simulink model "TestbedModel_v6"  (R2016a)
settings: Solver=ode23tb  StartTime=0.0  StopTime=20  RelTol=1e-3
undefined symbols (not defined in the file): K, Ki, Kp, magnitude, rev_comms_sink, tau
libraries: DAEMOT_Lib x4
(part 2 of 4)

== system TestbedModel_v6/Air Vehicle ==
  In1 : Inport
  In2 : Inport  Port=2
  Bus Creator2 : BusCreator  Inputs=4
  Bus Selector2 : BusSelector  OutputSignals=aspeed,torque
  Data_Sink : Subsystem  LoadFcn=|  InitFcn=|  mask(Data Sink){}
      LoadFcn=|
      | h      = get_param(gcb,'handle');   % Get block handle                           
      | hblock = get(h);     % Parse out handles structure
      | 
      | str = [hblock.Path(numel(bdroot)+2:end), hblock.Name];
      | str(~ismember(str,['A':'Z' 'a':'z' '0':'9' '_'])) = '';                     
      | set_param([gcb, '/global_data_goto'],'GotoTag',['gdata_',str]);
      |                                
      |                                                                                  
      | clear h hblock str
      InitFcn=|
      | h      = get_param(gcb,'handle');   % Get block handle                           
      | hblock = get(h);     % Parse out handles structure
      | 
      | str = [hblock.Path(numel(bdroot)+2:end), hblock.Name];
      | str(~ismember(str,['A':'Z' 'a':'z' '0':'9' '_'])) = '';                     
      | set_param([gcb, '/global_data_goto'],'GotoTag',['gdata_',str]);
      |                                
      |                                                                                  
      | clear h hblock str
      mask help:
      | Input to this block should be a bus signal with named signals.
      |
      | Bus signals sent to this block will be read by the Data Manager.
      | The Data Manager will handle the global routing of signals.
      |
      | This block should be placed under the mask of components.
      settings: CopyFcn=|
      | h      = get_param(gcb,'handle');   % Get block handle
      | hblock = get(h);     % Parse out handles structure
      | 
      | str = [hblock.Path(numel(bdroot)+2:end), hblock.Name];
      | str(~ismember(str,['A':'Z' 'a':'z' '0':'9' '_'])) = '';
      | set_param([gcb, '/global_data_goto'],'GotoTag',['gdata_',str]);
      | 
      | 
      | clear h hblock str
      settings: NameChangeFcn=|
      | h      = get_param(gcb,'handle');   % Get block handle
      | hblock = get(h);     % Parse out handles structure
      | 
      | str = [hblock.Path(numel(bdroot)+2:end), hblock.Name];
      | str(~ismember(str,['A':'Z' 'a':'z' '0':'9' '_'])) = '';
      | set_param([gcb, '/global_data_goto'],'GotoTag',['gdata_',str]);
      | 
      | 
      | clear h hblock str
      mask Display: text(0.25,0.5,'Data Sink')
  Fcn : Fcn  Expr=u(1)*cos(u(2))
  Fcn1 : Fcn  Expr=u(1)*sin(u(2))
  Integrator : Integrator  InitialCondition=v_initial
  Mux : Mux  Inputs=2
  Property : Subsystem
  Sink1 : Subsystem  LoadFcn=rev_comms_sink();  InitFcn=rev_comms_sink();  mask(Sink){}
      mask help: Used for sending data to the upstream component.
      settings: CopyFcn=rev_comms_sink();  NameChangeFcn=rev_comms_sink();
      mask Display: text(0.25,0.5,'Sink')
  Terminator1 : Terminator
  speed : MATLAB Function  TreatAsAtomicUnit=on
  wires:
  Property/1(Props) -> speed/3(props)
  Integrator/1 -> [v], Property/1(v), speed/1(v)
  [tau] -> Sink1/1(In1)
  Bus Selector2/1 -> [omega]  "<aspeed>"
  In1/1 -> Bus Selector2/1
  Bus Selector2/2 -> Terminator1/1  "<torque>"
  [v] -> Bus Creator2/2  "Vehicle Speed [m_s]"
  Bus Creator2/1 -> Data_Sink/1(" ")
  [tau] -> Bus Creator2/1  "Load Torque [Nm]"
  [omega] -> speed/2(omega), Property/2(w)
  speed/1(v_dot) -> Integrator/1
  speed/2(tau) -> [tau]
  [theta] -> speed/4(theta)
  Fcn/1 -> Bus Creator2/3  "Lateral Speed [m_s]"
  Fcn1/1 -> Bus Creator2/4  "Vertical Speed [m_s]"
  Mux/1 -> Fcn1/1, Fcn/1
  [v] -> Mux/1
  [theta] -> Mux/2
  In2/1 -> [theta]

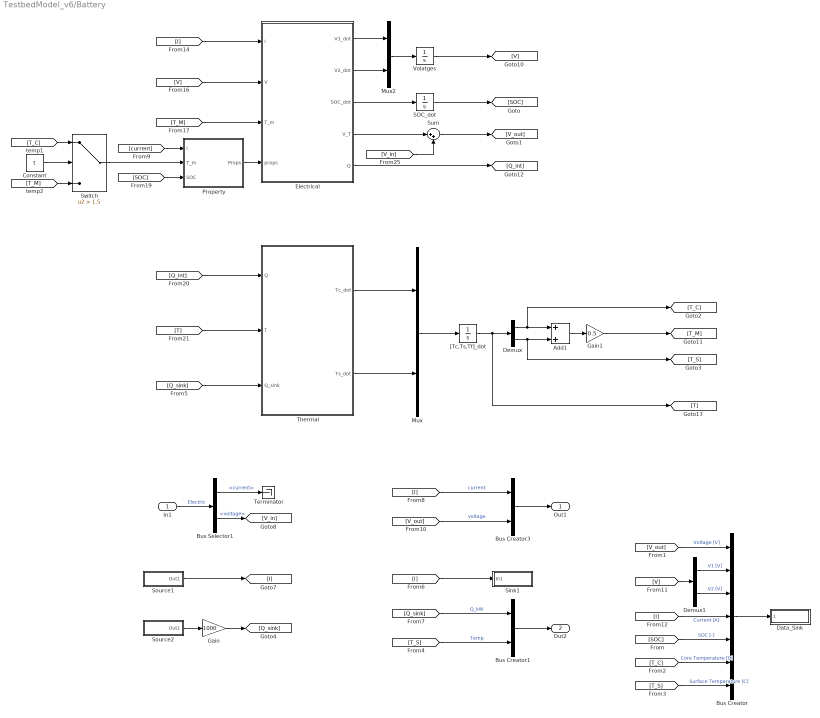
== system TestbedModel_v6/Battery ==
  In1 : Inport
  Add1 : Sum
  Bus Creator : BusCreator  Inputs=7
  Bus Creator1 : BusCreator  Inputs=2
  Bus Creator3 : BusCreator  Inputs=2
  Bus Selector1 : BusSelector  OutputSignals=current,voltage
  Constant : Constant  Value=t
  Data_Sink : Subsystem  LoadFcn=|  InitFcn=|  mask(Data Sink){}
      LoadFcn=|
      | h      = get_param(gcb,'handle');   % Get block handle                           
      | hblock = get(h);     % Parse out handles structure
      | 
      | str = [hblock.Path(numel(bdroot)+2:end), hblock.Name];
      | str(~ismember(str,['A':'Z' 'a':'z' '0':'9' '_'])) = '';                     
      | set_param([gcb, '/global_data_goto'],'GotoTag',['gdata_',str]);
      |                                
      |                                                                                  
      | clear h hblock str
      InitFcn=|
      | h      = get_param(gcb,'handle');   % Get block handle                           
      | hblock = get(h);     % Parse out handles structure
      | 
      | str = [hblock.Path(numel(bdroot)+2:end), hblock.Name];
      | str(~ismember(str,['A':'Z' 'a':'z' '0':'9' '_'])) = '';                     
      | set_param([gcb, '/global_data_goto'],'GotoTag',['gdata_',str]);
      |                                
      |                                                                                  
      | clear h hblock str
      mask help:
      | Input to this block should be a bus signal with named signals.
      |
      | Bus signals sent to this block will be read by the Data Manager.
      | The Data Manager will handle the global routing of signals.
      |
      | This block should be placed under the mask of components.
      settings: CopyFcn=|
      | h      = get_param(gcb,'handle');   % Get block handle
      | hblock = get(h);     % Parse out handles structure
      | 
      | str = [hblock.Path(numel(bdroot)+2:end), hblock.Name];
      | str(~ismember(str,['A':'Z' 'a':'z' '0':'9' '_'])) = '';
      | set_param([gcb, '/global_data_goto'],'GotoTag',['gdata_',str]);
      | 
      | 
      | clear h hblock str
      settings: NameChangeFcn=|
      | h      = get_param(gcb,'handle');   % Get block handle
      | hblock = get(h);     % Parse out handles structure
      | 
      | str = [hblock.Path(numel(bdroot)+2:end), hblock.Name];
      | str(~ismember(str,['A':'Z' 'a':'z' '0':'9' '_'])) = '';
      | set_param([gcb, '/global_data_goto'],'GotoTag',['gdata_',str]);
      | 
      | 
      | clear h hblock str
      mask Display: text(0.25,0.5,'Data Sink')
  Demux : Demux  Outputs=2
  Demux1 : Demux  Outputs=2
  Electrical : MATLAB Function  TreatAsAtomicUnit=on
  Gain : Gain  Gain=1000
  Gain1 : Gain  Gain=0.5
  Mux : Mux  Inputs=2
  Mux2 : Mux  Inputs=2
  Property : Subsystem
  SOC_dot : Integrator  InitialCondition=SOC_initial
  Sink1 : Subsystem  LoadFcn=rev_comms_sink();  InitFcn=rev_comms_sink();  mask(Sink){}
      mask help: Used for sending data to the upstream component.
      settings: CopyFcn=rev_comms_sink();  NameChangeFcn=rev_comms_sink();
      mask Display: text(0.25,0.5,'Sink')
  Source1 : Subsystem  mask(Source){}
      mask help: Used for receiving data from the downstream component.
      mask init:
      | n_src = gcb;
      | n_src = str2num(n_src(end));
      | try
      |     rev_comms_source(n_src);
      | catch
      | 
      | end
      mask Display: text(0.25,0.5,'Source')
  Source2 : Subsystem  mask(Source){}
      mask help: Used for receiving data from the downstream component.
      mask init:
      | n_src = gcb;
      | n_src = str2num(n_src(end));
      | try
      |     rev_comms_source(n_src);
      | catch
      | 
      | end
      mask Display: text(0.25,0.5,'Source')
  Sum : Sum  Inputs=|++
  Switch : Switch  Criteria=u2 > Threshold  Threshold=1.5
  Terminator : Terminator
  Thermal : MATLAB Function  TreatAsAtomicUnit=on
  Volatges : Integrator  InitialCondition=RC_initial
  "[Tc,Ts,Tf]_dot" : Integrator  InitialCondition=[Tc_initial, Ts_initial]
  Out1 : Outport
  Out2 : Outport  Port=2
  wires:
  Gain/1 -> [Q_sink]
  [Q_sink] -> Bus Creator1/1  "Q_kW"
  [T_S] -> Bus Creator1/2  "Temp"
  Bus Creator1/1 -> Out2/1
  Source1/1(Out1) -> [I]
  [I] -> Sink1/1(In1)
  Source2/1(Out1) -> Gain/1
  [Q_sink] -> Thermal/3(Q_sink)
  Thermal/2(Ts_dot) -> Mux/2
  Thermal/1(Tc_dot) -> Mux/1
  [T] -> Thermal/2(T)
  [Q_int] -> Thermal/1(Q)
  [SOC] -> Property/3(SOC)
  Bus Creator/1 -> Data_Sink/1(" ")
  Gain1/1 -> [T_M]
  [current] -> Property/1(I)
  [V_out] -> Bus Creator3/2  "voltage"
  Bus Selector1/2 -> [V_in]  "<voltage>"
  Bus Selector1/1 -> Terminator/1  "<current>"
  [I] -> Bus Creator3/1  "current"
  Bus Creator3/1 -> Out1/1
  In1/1 -> Bus Selector1/1  "Electric"
  [T_S] -> Bus Creator/7  "Surface Temperature [C]"
  [T_C] -> Bus Creator/6  "Core Temperature [C]"
  [V_out] -> Bus Creator/1  "Voltage [V]"
  [SOC] -> Bus Creator/5  "SOC [-]"
  Mux/1 -> "[Tc,Ts,Tf]_dot"/1
  Add1/1 -> Gain1/1
  Volatges/1 -> [V]
  SOC_dot/1 -> [SOC]
  "[Tc,Ts,Tf]_dot"/1 -> Demux/1, [T]
  Demux/1 -> Add1/1, [T_C]
  Demux/2 -> Add1/2, [T_S]
  Mux2/1 -> Volatges/1
  [I] -> Electrical/1(I)
  [T_M] -> Electrical/3(T_m)
  [V] -> Electrical/2(V)
  Property/1(Props) -> Electrical/4(props)
  Electrical/5(Q) -> [Q_int]
  [V_in] -> Sum/2
  Electrical/4(V_T) -> Sum/1
  Sum/1 -> [V_out]
  Electrical/3(SOC_dot) -> SOC_dot/1
  Electrical/1(V1_dot) -> Mux2/1
  Electrical/2(V2_dot) -> Mux2/2
  Constant/1 -> Switch/2
  [T_C] -> Switch/1
  [T_M] -> Switch/3
  Switch/1 -> Property/2(T_m)
  Demux1/2 -> Bus Creator/3  "V2 [V]"
  Demux1/1 -> Bus Creator/2  "V1 [V]"
  [V] -> Demux1/1
  [I] -> Bus Creator/4  "Current [A]"

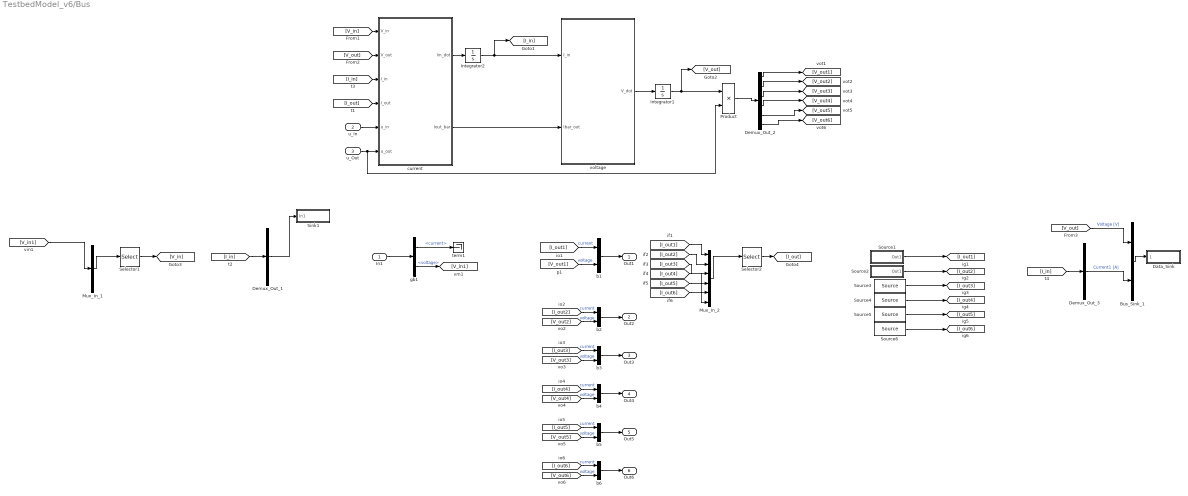
== system TestbedModel_v6/Bus ==
  In1 : Inport
  u_In : Inport  Port=2
  u_Out : Inport  Port=3
  Bus_Sink_1 : BusCreator  Inputs=2
  Data_Sink : Subsystem  LoadFcn=|  InitFcn=|  mask(Data Sink){}
      LoadFcn=|
      | h      = get_param(gcb,'handle');   % Get block handle                           
      | hblock = get(h);     % Parse out handles structure
      | 
      | str = [hblock.Path(numel(bdroot)+2:end), hblock.Name];
      | str(~ismember(str,['A':'Z' 'a':'z' '0':'9' '_'])) = '';                     
      | set_param([gcb, '/global_data_goto'],'GotoTag',['gdata_',str]);
      |                                
      |                                                                                  
      | clear h hblock str
      InitFcn=|
      | h      = get_param(gcb,'handle');   % Get block handle                           
      | hblock = get(h);     % Parse out handles structure
      | 
      | str = [hblock.Path(numel(bdroot)+2:end), hblock.Name];
      | str(~ismember(str,['A':'Z' 'a':'z' '0':'9' '_'])) = '';                     
      | set_param([gcb, '/global_data_goto'],'GotoTag',['gdata_',str]);
      |                                
      |                                                                                  
      | clear h hblock str
      mask help:
      | Input to this block should be a bus signal with named signals.
      |
      | Bus signals sent to this block will be read by the Data Manager.
      | The Data Manager will handle the global routing of signals.
      |
      | This block should be placed under the mask of components.
      settings: CopyFcn=|
      | h      = get_param(gcb,'handle');   % Get block handle
      | hblock = get(h);     % Parse out handles structure
      | 
      | str = [hblock.Path(numel(bdroot)+2:end), hblock.Name];
      | str(~ismember(str,['A':'Z' 'a':'z' '0':'9' '_'])) = '';
      | set_param([gcb, '/global_data_goto'],'GotoTag',['gdata_',str]);
      | 
      | 
      | clear h hblock str
      settings: NameChangeFcn=|
      | h      = get_param(gcb,'handle');   % Get block handle
      | hblock = get(h);     % Parse out handles structure
      | 
      | str = [hblock.Path(numel(bdroot)+2:end), hblock.Name];
      | str(~ismember(str,['A':'Z' 'a':'z' '0':'9' '_'])) = '';
      | set_param([gcb, '/global_data_goto'],'GotoTag',['gdata_',str]);
      | 
      | 
      | clear h hblock str
      mask Display: text(0.25,0.5,'Data Sink')
  Demux_Out_1 : Demux  Outputs=1
  Demux_Out_2 : Demux  Outputs=6
  Demux_Out_3 : Demux  Outputs=1
  Integrator1 : Integrator  InitialCondition=V_initial
  Integrator2 : Integrator  InitialCondition=I_initial*ones(Num_In,1)
  Mux_In_1 : Mux  Inputs=1
  Mux_In_2 : Mux  Inputs=6
  Product : Product
  Selector1 : Selector  InputPortWidth=1  IndexOptions=Index vector (dialog)  Indices=[1 ]  OutputSizes=1
  Selector2 : Selector  InputPortWidth=6  IndexOptions=Index vector (dialog)  Indices=[1 2 3 4 5 6 ]  OutputSizes=1
  Sink1 : Subsystem  LoadFcn=rev_comms_sink();  InitFcn=rev_comms_sink();  mask(Sink){}
      mask help: Used for sending data to the upstream component.
      settings: CopyFcn=rev_comms_sink();  NameChangeFcn=rev_comms_sink();
      mask Display: text(0.25,0.5,'Sink')
  Source1 : Subsystem  mask(Source){}
      mask help: Used for receiving data from the downstream component.
      mask init:
      | n_src = gcb;
      | n_src = str2num(n_src(end));
      | try
      |     rev_comms_source(n_src);
      | catch
      | 
      | end
      mask Display: text(0.25,0.5,'Source')
  Source2 : Subsystem  mask(Source){}
      mask help: Used for receiving data from the downstream component.
      mask init:
      | n_src = gcb;
      | n_src = str2num(n_src(end));
      | try
      |     rev_comms_source(n_src);
      | catch
      | 
      | end
      mask Display: text(0.25,0.5,'Source')
  Source{3..6} (4 alike) : DAEMOT_Lib/Support Functions/Source
  b{1..6} (6 alike) : BusCreator  Inputs=2
  current : MATLAB Function  TreatAsAtomicUnit=on
  gb1 : BusSelector  OutputSignals=current,voltage
  term1 : Terminator
  voltage : MATLAB Function  TreatAsAtomicUnit=on
  Out1 : Outport
  Out2 : Outport  Port=2
  Out3 : Outport  Port=3
  Out4 : Outport  Port=4
  Out5 : Outport  Port=5
  Out6 : Outport  Port=6
  wires:
  Demux_Out_2/2 -> [V_out2]
  [I_out2] -> Mux_In_2/2
  Source2/1(Out1) -> [I_out2]
  b2/1 -> Out2/1
  [V_out2] -> b2/2  "voltage"
  [I_out2] -> b2/1  "current"
  [V_out] -> Bus_Sink_1/1  "Voltage [V]"
  Selector2/1 -> [I_out]
  [I_out] -> current/4(I_out)
  Selector1/1 -> [V_in]
  [V_in] -> current/1(V_in)
  Product/1 -> Demux_Out_2/1
  current/2(Iout_bar) -> voltage/2(Ibar_out)
  u_Out/1 -> current/6(u_out), Product/2
  b1/1 -> Out1/1
  Source1/1(Out1) -> [I_out1]
  [I_out1] -> b1/1  "current"
  [V_out1] -> b1/2  "voltage"
  Mux_In_2/1 -> Selector2/1
  [I_out1] -> Mux_In_2/1
  Bus_Sink_1/1 -> Data_Sink/1(" ")
  Demux_Out_2/1 -> [V_out1]
  u_In/1 -> current/5(u_in)
  [I_in] -> current/3(I_in)
  current/1(Iin_dot) -> Integrator2/1
  Mux_In_1/1 -> Selector1/1
  [V_out] -> current/2(V_out)
  Integrator1/1 -> [V_out], Product/1
  voltage/1(V_dot) -> Integrator1/1
  Integrator2/1 -> [I_in], voltage/1(I_in)
  [I_in] -> Demux_Out_1/1
  In1/1 -> gb1/1
  gb1/1 -> term1/1  "<current>"
  gb1/2 -> [V_in1]  "<voltage>"
  [V_in1] -> Mux_In_1/1
  Demux_Out_1/1 -> Sink1/1(In1)
  [I_in] -> Demux_Out_3/1
  Demux_Out_3/1 -> Bus_Sink_1/2  "Current1 [A]"
  [I_out3] -> b3/1  "current"
  [V_out3] -> b3/2  "voltage"
  b3/1 -> Out3/1
  Source3/1 -> [I_out3]
  [I_out3] -> Mux_In_2/3
  Demux_Out_2/3 -> [V_out3]
  [I_out4] -> b4/1  "current"
  [V_out4] -> b4/2  "voltage"
  b4/1 -> Out4/1
  Source4/1 -> [I_out4]
  [I_out4] -> Mux_In_2/4
  Demux_Out_2/4 -> [V_out4]
  [I_out5] -> b5/1  "current"
  [V_out5] -> b5/2  "voltage"
  b5/1 -> Out5/1
  Source5/1 -> [I_out5]
  [I_out5] -> Mux_In_2/5
  Demux_Out_2/5 -> [V_out5]
  [I_out6] -> b6/1  "current"
  [V_out6] -> b6/2  "voltage"
  b6/1 -> Out6/1
  Source6/1 -> [I_out6]
  [I_out6] -> Mux_In_2/6
  Demux_Out_2/6 -> [V_out6]

== system TestbedModel_v6/Capacitor ==
  In1 : Inport
  Bus Creator1 : BusCreator  Inputs=1
  Bus Creator3 : BusCreator  Inputs=2
  Bus Selector1 : BusSelector  OutputSignals=current,voltage
  Data_Sink : Subsystem  LoadFcn=|  InitFcn=|  mask(Data Sink){}
      LoadFcn=|
      | h      = get_param(gcb,'handle');   % Get block handle                           
      | hblock = get(h);     % Parse out handles structure
      | 
      | str = [hblock.Path(numel(bdroot)+2:end), hblock.Name];
      | str(~ismember(str,['A':'Z' 'a':'z' '0':'9' '_'])) = '';                     
      | set_param([gcb, '/global_data_goto'],'GotoTag',['gdata_',str]);
      |                                
      |                                                                                  
      | clear h hblock str
      InitFcn=|
      | h      = get_param(gcb,'handle');   % Get block handle                           
      | hblock = get(h);     % Parse out handles structure
      | 
      | str = [hblock.Path(numel(bdroot)+2:end), hblock.Name];
      | str(~ismember(str,['A':'Z' 'a':'z' '0':'9' '_'])) = '';                     
      | set_param([gcb, '/global_data_goto'],'GotoTag',['gdata_',str]);
      |                                
      |                                                                                  
      | clear h hblock str
      mask help:
      | Input to this block should be a bus signal with named signals.
      |
      | Bus signals sent to this block will be read by the Data Manager.
      | The Data Manager will handle the global routing of signals.
      |
      | This block should be placed under the mask of components.
      settings: CopyFcn=|
      | h      = get_param(gcb,'handle');   % Get block handle
      | hblock = get(h);     % Parse out handles structure
      | 
      | str = [hblock.Path(numel(bdroot)+2:end), hblock.Name];
      | str(~ismember(str,['A':'Z' 'a':'z' '0':'9' '_'])) = '';
      | set_param([gcb, '/global_data_goto'],'GotoTag',['gdata_',str]);
      | 
      | 
      | clear h hblock str
      settings: NameChangeFcn=|
      | h      = get_param(gcb,'handle');   % Get block handle
      | hblock = get(h);     % Parse out handles structure
      | 
      | str = [hblock.Path(numel(bdroot)+2:end), hblock.Name];
      | str(~ismember(str,['A':'Z' 'a':'z' '0':'9' '_'])) = '';
      | set_param([gcb, '/global_data_goto'],'GotoTag',['gdata_',str]);
      | 
      | 
      | clear h hblock str
      mask Display: text(0.25,0.5,'Data Sink')
  Integrator2 : Integrator  InitialCondition=V_initial
  Sink1 : Subsystem  LoadFcn=rev_comms_sink();  InitFcn=rev_comms_sink();  mask(Sink){}
      mask help: Used for sending data to the upstream component.
      settings: CopyFcn=rev_comms_sink();  NameChangeFcn=rev_comms_sink();
      mask Display: text(0.25,0.5,'Sink')
  Source1 : Subsystem  mask(Source){}
      mask help: Used for receiving data from the downstream component.
      mask init:
      | n_src = gcb;
      | n_src = str2num(n_src(end));
      | try
      |     rev_comms_source(n_src);
      | catch
      | 
      | end
      mask Display: text(0.25,0.5,'Source')
  Terminator : Terminator
  Voltage : MATLAB Function  TreatAsAtomicUnit=on
  Out1 : Outport
  wires:
  Source1/1(Out1) -> [Current_out]
  Bus Creator1/1 -> Data_Sink/1(" ")
  [V] -> Bus Creator1/1  "Voltage [V]"
  [Current_in] -> Voltage/1(I_in)
  Voltage/1(V_dot) -> Integrator2/1
  Bus Creator3/1 -> Out1/1
  [Current_out] -> Voltage/2(I_out)
  In1/1 -> Bus Selector1/1  "electric"
  [V] -> Sink1/1(In1)
  [V] -> Bus Creator3/2  "voltage"
  Bus Selector1/2 -> Terminator/1  "<voltage>"
  Bus Selector1/1 -> [Current_in]  "<current>"
  [Current_out] -> Bus Creator3/1  "current"
  Integrator2/1 -> [V]

== system TestbedModel_v6/Capacitor1 ==
  In1 : Inport
  Bus Creator1 : BusCreator  Inputs=1
  Bus Creator3 : BusCreator  Inputs=2
  Bus Selector1 : BusSelector  OutputSignals=current,voltage
  Data_Sink : Subsystem  LoadFcn=|  InitFcn=|  mask(Data Sink){}
      LoadFcn=|
      | h      = get_param(gcb,'handle');   % Get block handle                           
      | hblock = get(h);     % Parse out handles structure
      | 
      | str = [hblock.Path(numel(bdroot)+2:end), hblock.Name];
      | str(~ismember(str,['A':'Z' 'a':'z' '0':'9' '_'])) = '';                     
      | set_param([gcb, '/global_data_goto'],'GotoTag',['gdata_',str]);
      |                                
      |                                                                                  
      | clear h hblock str
      InitFcn=|
      | h      = get_param(gcb,'handle');   % Get block handle                           
      | hblock = get(h);     % Parse out handles structure
      | 
      | str = [hblock.Path(numel(bdroot)+2:end), hblock.Name];
      | str(~ismember(str,['A':'Z' 'a':'z' '0':'9' '_'])) = '';                     
      | set_param([gcb, '/global_data_goto'],'GotoTag',['gdata_',str]);
      |                                
      |                                                                                  
      | clear h hblock str
      mask help:
      | Input to this block should be a bus signal with named signals.
      |
      | Bus signals sent to this block will be read by the Data Manager.
      | The Data Manager will handle the global routing of signals.
      |
      | This block should be placed under the mask of components.
      settings: CopyFcn=|
      | h      = get_param(gcb,'handle');   % Get block handle
      | hblock = get(h);     % Parse out handles structure
      | 
      | str = [hblock.Path(numel(bdroot)+2:end), hblock.Name];
      | str(~ismember(str,['A':'Z' 'a':'z' '0':'9' '_'])) = '';
      | set_param([gcb, '/global_data_goto'],'GotoTag',['gdata_',str]);
      | 
      | 
      | clear h hblock str
      settings: NameChangeFcn=|
      | h      = get_param(gcb,'handle');   % Get block handle
      | hblock = get(h);     % Parse out handles structure
      | 
      | str = [hblock.Path(numel(bdroot)+2:end), hblock.Name];
      | str(~ismember(str,['A':'Z' 'a':'z' '0':'9' '_'])) = '';
      | set_param([gcb, '/global_data_goto'],'GotoTag',['gdata_',str]);
      | 
      | 
      | clear h hblock str
      mask Display: text(0.25,0.5,'Data Sink')
  Integrator2 : Integrator  InitialCondition=V_initial
  Sink1 : Subsystem  LoadFcn=rev_comms_sink();  InitFcn=rev_comms_sink();  mask(Sink){}
      mask help: Used for sending data to the upstream component.
      settings: CopyFcn=rev_comms_sink();  NameChangeFcn=rev_comms_sink();
      mask Display: text(0.25,0.5,'Sink')
  Source1 : Subsystem  mask(Source){}
      mask help: Used for receiving data from the downstream component.
      mask init:
      | n_src = gcb;
      | n_src = str2num(n_src(end));
      | try
      |     rev_comms_source(n_src);
      | catch
      | 
      | end
      mask Display: text(0.25,0.5,'Source')
  Terminator : Terminator
  Voltage : MATLAB Function  TreatAsAtomicUnit=on
  Out1 : Outport
  wires:
  Integrator2/1 -> [V]
  [Current_out] -> Bus Creator3/1  "current"
  Bus Selector1/1 -> [Current_in]  "<current>"
  Bus Selector1/2 -> Terminator/1  "<voltage>"
  [V] -> Bus Creator3/2  "voltage"
  [V] -> Sink1/1(In1)
  In1/1 -> Bus Selector1/1  "electric"
  [Current_out] -> Voltage/2(I_out)
  Bus Creator3/1 -> Out1/1
  Voltage/1(V_dot) -> Integrator2/1
  [Current_in] -> Voltage/1(I_in)
  [V] -> Bus Creator1/1  "Voltage [V]"
  Bus Creator1/1 -> Data_Sink/1(" ")
  Source1/1(Out1) -> [Current_out]

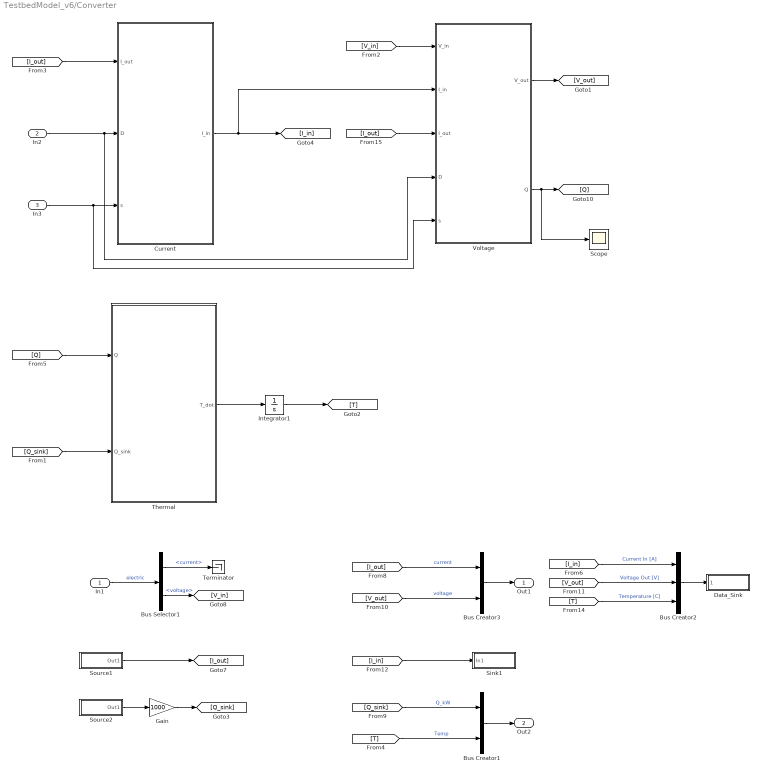
== system TestbedModel_v6/Converter ==
  In1 : Inport
  In2 : Inport  Port=2
  In3 : Inport  Port=3
  Bus Creator1 : BusCreator  Inputs=2
  Bus Creator2 : BusCreator  Inputs=3
  Bus Creator3 : BusCreator  Inputs=2
  Bus Selector1 : BusSelector  OutputSignals=current,voltage
  Current : MATLAB Function  TreatAsAtomicUnit=on
  Data_Sink : Subsystem  LoadFcn=|  InitFcn=|  mask(Data Sink){}
      LoadFcn=|
      | h      = get_param(gcb,'handle');   % Get block handle                           
      | hblock = get(h);     % Parse out handles structure
      | 
      | str = [hblock.Path(numel(bdroot)+2:end), hblock.Name];
      | str(~ismember(str,['A':'Z' 'a':'z' '0':'9' '_'])) = '';                     
      | set_param([gcb, '/global_data_goto'],'GotoTag',['gdata_',str]);
      |                                
      |                                                                                  
      | clear h hblock str
      InitFcn=|
      | h      = get_param(gcb,'handle');   % Get block handle                           
      | hblock = get(h);     % Parse out handles structure
      | 
      | str = [hblock.Path(numel(bdroot)+2:end), hblock.Name];
      | str(~ismember(str,['A':'Z' 'a':'z' '0':'9' '_'])) = '';                     
      | set_param([gcb, '/global_data_goto'],'GotoTag',['gdata_',str]);
      |                                
      |                                                                                  
      | clear h hblock str
      mask help:
      | Input to this block should be a bus signal with named signals.
      |
      | Bus signals sent to this block will be read by the Data Manager.
      | The Data Manager will handle the global routing of signals.
      |
      | This block should be placed under the mask of components.
      settings: CopyFcn=|
      | h      = get_param(gcb,'handle');   % Get block handle
      | hblock = get(h);     % Parse out handles structure
      | 
      | str = [hblock.Path(numel(bdroot)+2:end), hblock.Name];
      | str(~ismember(str,['A':'Z' 'a':'z' '0':'9' '_'])) = '';
      | set_param([gcb, '/global_data_goto'],'GotoTag',['gdata_',str]);
      | 
      | 
      | clear h hblock str
      settings: NameChangeFcn=|
      | h      = get_param(gcb,'handle');   % Get block handle
      | hblock = get(h);     % Parse out handles structure
      | 
      | str = [hblock.Path(numel(bdroot)+2:end), hblock.Name];
      | str(~ismember(str,['A':'Z' 'a':'z' '0':'9' '_'])) = '';
      | set_param([gcb, '/global_data_goto'],'GotoTag',['gdata_',str]);
      | 
      | 
      | clear h hblock str
      mask Display: text(0.25,0.5,'Data Sink')
  Gain : Gain  Gain=1000
  Integrator1 : Integrator  InitialCondition=T_initial
  Scope : Scope
  Sink1 : Subsystem  LoadFcn=rev_comms_sink();  InitFcn=rev_comms_sink();  mask(Sink){}
      mask help: Used for sending data to the upstream component.
      settings: CopyFcn=rev_comms_sink();  NameChangeFcn=rev_comms_sink();
      mask Display: text(0.25,0.5,'Sink')
  Source1 : Subsystem  mask(Source){}
      mask help: Used for receiving data from the downstream component.
      mask init:
      | n_src = gcb;
      | n_src = str2num(n_src(end));
      | try
      |     rev_comms_source(n_src);
      | catch
      | 
      | end
      mask Display: text(0.25,0.5,'Source')
  Source2 : Subsystem  mask(Source){}
      mask help: Used for receiving data from the downstream component.
      mask init:
      | n_src = gcb;
      | n_src = str2num(n_src(end));
      | try
      |     rev_comms_source(n_src);
      | catch
      | 
      | end
      mask Display: text(0.25,0.5,'Source')
  Terminator : Terminator
  Thermal : MATLAB Function  TreatAsAtomicUnit=on
  Voltage : MATLAB Function  TreatAsAtomicUnit=on
  Out1 : Outport
  Out2 : Outport  Port=2
  wires:
  Source2/1(Out1) -> Gain/1
  Voltage/2(Q) -> Scope/1, [Q]
  [I_out] -> Voltage/3(I_out)
  [T] -> Bus Creator2/3  "Temperature [C]"
  [I_in] -> Bus Creator2/1  "Current In [A]"
  [V_out] -> Bus Creator2/2  "Voltage Out [V]"
  Bus Creator2/1 -> Data_Sink/1(" ")
  Thermal/1(T_dot) -> Integrator1/1
  Integrator1/1 -> [T]
  [Q] -> Thermal/1(Q)
  [Q_sink] -> Thermal/2(Q_sink)
  In3/1 -> Current/3(s), Voltage/5(s)
  In2/1 -> Current/2(D), Voltage/4(D)
  Current/1(I_in) -> [I_in], Voltage/2(I_in)
  [I_out] -> Current/1(I_out)
  Voltage/1(V_out) -> [V_out]
  [V_in] -> Voltage/1(V_in)
  [I_out] -> Bus Creator3/1  "current"
  Source1/1(Out1) -> [I_out]
  Bus Selector1/1 -> Terminator/1  "<current>"
  Bus Selector1/2 -> [V_in]  "<voltage>"
  [V_out] -> Bus Creator3/2  "voltage"
  In1/1 -> Bus Selector1/1  "electric"
  Bus Creator3/1 -> Out1/1
  [I_in] -> Sink1/1(In1)
  Bus Creator1/1 -> Out2/1
  [T] -> Bus Creator1/2  "Temp"
  [Q_sink] -> Bus Creator1/1  "Q_kW"
  Gain/1 -> [Q_sink]

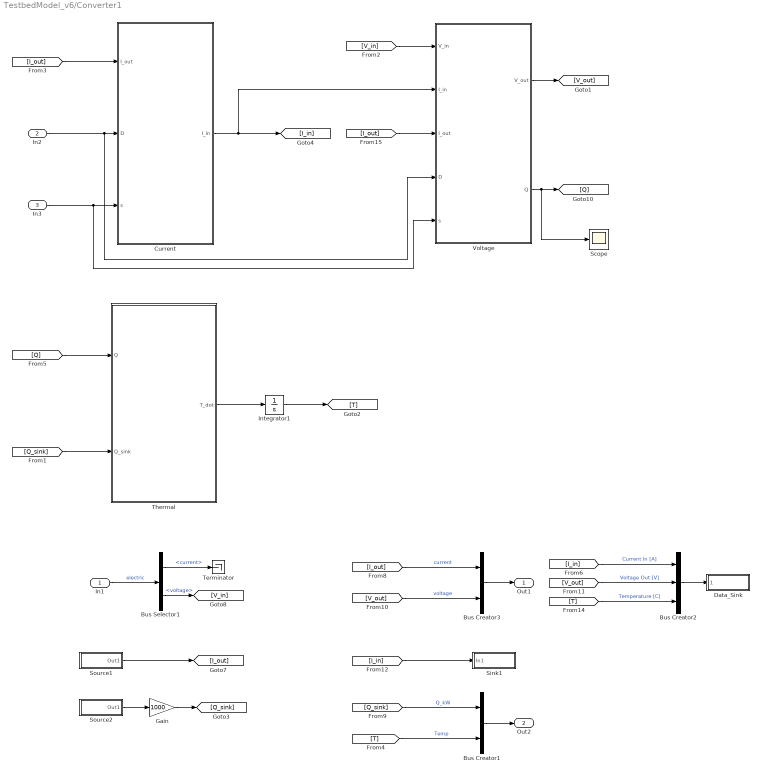
== system TestbedModel_v6/Converter1 ==
  In1 : Inport
  In2 : Inport  Port=2
  In3 : Inport  Port=3
  Bus Creator1 : BusCreator  Inputs=2
  Bus Creator2 : BusCreator  Inputs=3
  Bus Creator3 : BusCreator  Inputs=2
  Bus Selector1 : BusSelector  OutputSignals=current,voltage
  Current : MATLAB Function  TreatAsAtomicUnit=on
  Data_Sink : Subsystem  LoadFcn=|  InitFcn=|  mask(Data Sink){}
      LoadFcn=|
      | h      = get_param(gcb,'handle');   % Get block handle                           
      | hblock = get(h);     % Parse out handles structure
      | 
      | str = [hblock.Path(numel(bdroot)+2:end), hblock.Name];
      | str(~ismember(str,['A':'Z' 'a':'z' '0':'9' '_'])) = '';                     
      | set_param([gcb, '/global_data_goto'],'GotoTag',['gdata_',str]);
      |                                
      |                                                                                  
      | clear h hblock str
      InitFcn=|
      | h      = get_param(gcb,'handle');   % Get block handle                           
      | hblock = get(h);     % Parse out handles structure
      | 
      | str = [hblock.Path(numel(bdroot)+2:end), hblock.Name];
      | str(~ismember(str,['A':'Z' 'a':'z' '0':'9' '_'])) = '';                     
      | set_param([gcb, '/global_data_goto'],'GotoTag',['gdata_',str]);
      |                                
      |                                                                                  
      | clear h hblock str
      mask help:
      | Input to this block should be a bus signal with named signals.
      |
      | Bus signals sent to this block will be read by the Data Manager.
      | The Data Manager will handle the global routing of signals.
      |
      | This block should be placed under the mask of components.
      settings: CopyFcn=|
      | h      = get_param(gcb,'handle');   % Get block handle
      | hblock = get(h);     % Parse out handles structure
      | 
      | str = [hblock.Path(numel(bdroot)+2:end), hblock.Name];
      | str(~ismember(str,['A':'Z' 'a':'z' '0':'9' '_'])) = '';
      | set_param([gcb, '/global_data_goto'],'GotoTag',['gdata_',str]);
      | 
      | 
      | clear h hblock str
      settings: NameChangeFcn=|
      | h      = get_param(gcb,'handle');   % Get block handle
      | hblock = get(h);     % Parse out handles structure
      | 
      | str = [hblock.Path(numel(bdroot)+2:end), hblock.Name];
      | str(~ismember(str,['A':'Z' 'a':'z' '0':'9' '_'])) = '';
      | set_param([gcb, '/global_data_goto'],'GotoTag',['gdata_',str]);
      | 
      | 
      | clear h hblock str
      mask Display: text(0.25,0.5,'Data Sink')
  Gain : Gain  Gain=1000
  Integrator1 : Integrator  InitialCondition=T_initial
  Scope : Scope
  Sink1 : Subsystem  LoadFcn=rev_comms_sink();  InitFcn=rev_comms_sink();  mask(Sink){}
      mask help: Used for sending data to the upstream component.
      settings: CopyFcn=rev_comms_sink();  NameChangeFcn=rev_comms_sink();
      mask Display: text(0.25,0.5,'Sink')
  Source1 : Subsystem  mask(Source){}
      mask help: Used for receiving data from the downstream component.
      mask init:
      | n_src = gcb;
      | n_src = str2num(n_src(end));
      | try
      |     rev_comms_source(n_src);
      | catch
      | 
      | end
      mask Display: text(0.25,0.5,'Source')
  Source2 : Subsystem  mask(Source){}
      mask help: Used for receiving data from the downstream component.
      mask init:
      | n_src = gcb;
      | n_src = str2num(n_src(end));
      | try
      |     rev_comms_source(n_src);
      | catch
      | 
      | end
      mask Display: text(0.25,0.5,'Source')
  Terminator : Terminator
  Thermal : MATLAB Function  TreatAsAtomicUnit=on
  Voltage : MATLAB Function  TreatAsAtomicUnit=on
  Out1 : Outport
  Out2 : Outport  Port=2
  wires:
  Gain/1 -> [Q_sink]
  [Q_sink] -> Bus Creator1/1  "Q_kW"
  [T] -> Bus Creator1/2  "Temp"
  Bus Creator1/1 -> Out2/1
  [I_in] -> Sink1/1(In1)
  Bus Creator3/1 -> Out1/1
  In1/1 -> Bus Selector1/1  "electric"
  [V_out] -> Bus Creator3/2  "voltage"
  Bus Selector1/2 -> [V_in]  "<voltage>"
  Bus Selector1/1 -> Terminator/1  "<current>"
  Source1/1(Out1) -> [I_out]
  [I_out] -> Bus Creator3/1  "current"
  [V_in] -> Voltage/1(V_in)
  Voltage/1(V_out) -> [V_out]
  [I_out] -> Current/1(I_out)
  Current/1(I_in) -> Voltage/2(I_in), [I_in]
  In2/1 -> Voltage/4(D), Current/2(D)
  In3/1 -> Voltage/5(s), Current/3(s)
  [Q_sink] -> Thermal/2(Q_sink)
  [Q] -> Thermal/1(Q)
  Integrator1/1 -> [T]
  Thermal/1(T_dot) -> Integrator1/1
  Bus Creator2/1 -> Data_Sink/1(" ")
  [V_out] -> Bus Creator2/2  "Voltage Out [V]"
  [I_in] -> Bus Creator2/1  "Current In [A]"
  [T] -> Bus Creator2/3  "Temperature [C]"
  [I_out] -> Voltage/3(I_out)
  Voltage/2(Q) -> [Q], Scope/1
  Source2/1(Out1) -> Gain/1

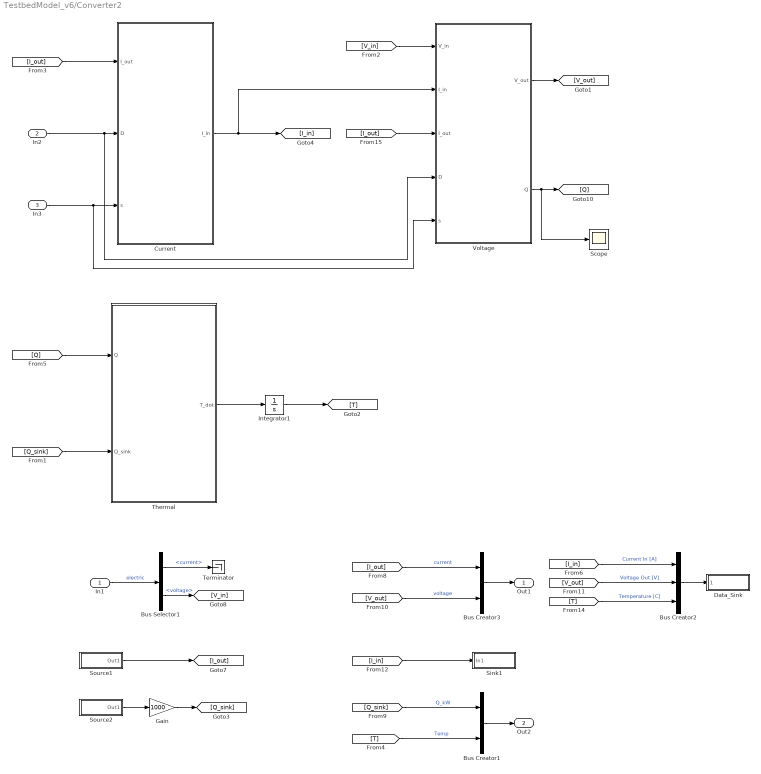
== system TestbedModel_v6/Converter2 ==
  In1 : Inport
  In2 : Inport  Port=2
  In3 : Inport  Port=3
  Bus Creator1 : BusCreator  Inputs=2
  Bus Creator2 : BusCreator  Inputs=3
  Bus Creator3 : BusCreator  Inputs=2
  Bus Selector1 : BusSelector  OutputSignals=current,voltage
  Current : MATLAB Function  TreatAsAtomicUnit=on
  Data_Sink : Subsystem  LoadFcn=|  InitFcn=|  mask(Data Sink){}
      LoadFcn=|
      | h      = get_param(gcb,'handle');   % Get block handle                           
      | hblock = get(h);     % Parse out handles structure
      | 
      | str = [hblock.Path(numel(bdroot)+2:end), hblock.Name];
      | str(~ismember(str,['A':'Z' 'a':'z' '0':'9' '_'])) = '';                     
      | set_param([gcb, '/global_data_goto'],'GotoTag',['gdata_',str]);
      |                                
      |                                                                                  
      | clear h hblock str
      InitFcn=|
      | h      = get_param(gcb,'handle');   % Get block handle                           
      | hblock = get(h);     % Parse out handles structure
      | 
      | str = [hblock.Path(numel(bdroot)+2:end), hblock.Name];
      | str(~ismember(str,['A':'Z' 'a':'z' '0':'9' '_'])) = '';                     
      | set_param([gcb, '/global_data_goto'],'GotoTag',['gdata_',str]);
      |                                
      |                                                                                  
      | clear h hblock str
      mask help:
      | Input to this block should be a bus signal with named signals.
      |
      | Bus signals sent to this block will be read by the Data Manager.
      | The Data Manager will handle the global routing of signals.
      |
      | This block should be placed under the mask of components.
      settings: CopyFcn=|
      | h      = get_param(gcb,'handle');   % Get block handle
      | hblock = get(h);     % Parse out handles structure
      | 
      | str = [hblock.Path(numel(bdroot)+2:end), hblock.Name];
      | str(~ismember(str,['A':'Z' 'a':'z' '0':'9' '_'])) = '';
      | set_param([gcb, '/global_data_goto'],'GotoTag',['gdata_',str]);
      | 
      | 
      | clear h hblock str
      settings: NameChangeFcn=|
      | h      = get_param(gcb,'handle');   % Get block handle
      | hblock = get(h);     % Parse out handles structure
      | 
      | str = [hblock.Path(numel(bdroot)+2:end), hblock.Name];
      | str(~ismember(str,['A':'Z' 'a':'z' '0':'9' '_'])) = '';
      | set_param([gcb, '/global_data_goto'],'GotoTag',['gdata_',str]);
      | 
      | 
      | clear h hblock str
      mask Display: text(0.25,0.5,'Data Sink')
  Gain : Gain  Gain=1000
  Integrator1 : Integrator  InitialCondition=T_initial
  Scope : Scope
  Sink1 : Subsystem  LoadFcn=rev_comms_sink();  InitFcn=rev_comms_sink();  mask(Sink){}
      mask help: Used for sending data to the upstream component.
      settings: CopyFcn=rev_comms_sink();  NameChangeFcn=rev_comms_sink();
      mask Display: text(0.25,0.5,'Sink')
  Source1 : Subsystem  mask(Source){}
      mask help: Used for receiving data from the downstream component.
      mask init:
      | n_src = gcb;
      | n_src = str2num(n_src(end));
      | try
      |     rev_comms_source(n_src);
      | catch
      | 
      | end
      mask Display: text(0.25,0.5,'Source')
  Source2 : Subsystem  mask(Source){}
      mask help: Used for receiving data from the downstream component.
      mask init:
      | n_src = gcb;
      | n_src = str2num(n_src(end));
      | try
      |     rev_comms_source(n_src);
      | catch
      | 
      | end
      mask Display: text(0.25,0.5,'Source')
  Terminator : Terminator
  Thermal : MATLAB Function  TreatAsAtomicUnit=on
  Voltage : MATLAB Function  TreatAsAtomicUnit=on
  Out1 : Outport
  Out2 : Outport  Port=2
  wires:
  Source2/1(Out1) -> Gain/1
  Voltage/2(Q) -> Scope/1, [Q]
  [I_out] -> Voltage/3(I_out)
  [T] -> Bus Creator2/3  "Temperature [C]"
  [I_in] -> Bus Creator2/1  "Current In [A]"
  [V_out] -> Bus Creator2/2  "Voltage Out [V]"
  Bus Creator2/1 -> Data_Sink/1(" ")
  Thermal/1(T_dot) -> Integrator1/1
  Integrator1/1 -> [T]
  [Q] -> Thermal/1(Q)
  [Q_sink] -> Thermal/2(Q_sink)
  In3/1 -> Current/3(s), Voltage/5(s)
  In2/1 -> Current/2(D), Voltage/4(D)
  Current/1(I_in) -> [I_in], Voltage/2(I_in)
  [I_out] -> Current/1(I_out)
  Voltage/1(V_out) -> [V_out]
  [V_in] -> Voltage/1(V_in)
  [I_out] -> Bus Creator3/1  "current"
  Source1/1(Out1) -> [I_out]
  Bus Selector1/1 -> Terminator/1  "<current>"
  Bus Selector1/2 -> [V_in]  "<voltage>"
  [V_out] -> Bus Creator3/2  "voltage"
  In1/1 -> Bus Selector1/1  "electric"
  Bus Creator3/1 -> Out1/1
  [I_in] -> Sink1/1(In1)
  Bus Creator1/1 -> Out2/1
  [T] -> Bus Creator1/2  "Temp"
  [Q_sink] -> Bus Creator1/1  "Q_kW"
  Gain/1 -> [Q_sink]

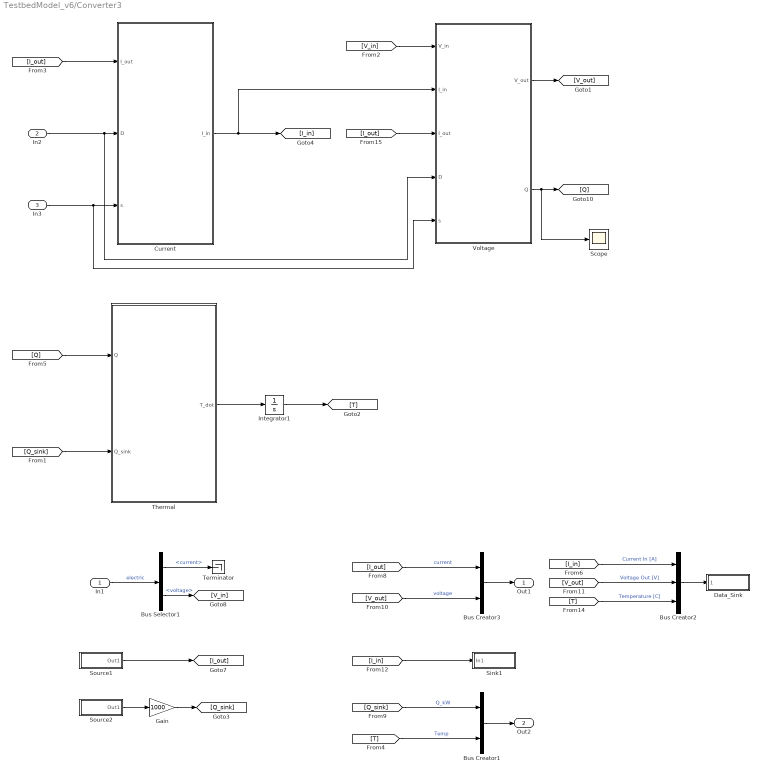
== system TestbedModel_v6/Converter3 ==
  In1 : Inport
  In2 : Inport  Port=2
  In3 : Inport  Port=3
  Bus Creator1 : BusCreator  Inputs=2
  Bus Creator2 : BusCreator  Inputs=3
  Bus Creator3 : BusCreator  Inputs=2
  Bus Selector1 : BusSelector  OutputSignals=current,voltage
  Current : MATLAB Function  TreatAsAtomicUnit=on
  Data_Sink : Subsystem  LoadFcn=|  InitFcn=|  mask(Data Sink){}
      LoadFcn=|
      | h      = get_param(gcb,'handle');   % Get block handle                           
      | hblock = get(h);     % Parse out handles structure
      | 
      | str = [hblock.Path(numel(bdroot)+2:end), hblock.Name];
      | str(~ismember(str,['A':'Z' 'a':'z' '0':'9' '_'])) = '';                     
      | set_param([gcb, '/global_data_goto'],'GotoTag',['gdata_',str]);
      |                                
      |                                                                                  
      | clear h hblock str
      InitFcn=|
      | h      = get_param(gcb,'handle');   % Get block handle                           
      | hblock = get(h);     % Parse out handles structure
      | 
      | str = [hblock.Path(numel(bdroot)+2:end), hblock.Name];
      | str(~ismember(str,['A':'Z' 'a':'z' '0':'9' '_'])) = '';                     
      | set_param([gcb, '/global_data_goto'],'GotoTag',['gdata_',str]);
      |                                
      |                                                                                  
      | clear h hblock str
      mask help:
      | Input to this block should be a bus signal with named signals.
      |
      | Bus signals sent to this block will be read by the Data Manager.
      | The Data Manager will handle the global routing of signals.
      |
      | This block should be placed under the mask of components.
      settings: CopyFcn=|
      | h      = get_param(gcb,'handle');   % Get block handle
      | hblock = get(h);     % Parse out handles structure
      | 
      | str = [hblock.Path(numel(bdroot)+2:end), hblock.Name];
      | str(~ismember(str,['A':'Z' 'a':'z' '0':'9' '_'])) = '';
      | set_param([gcb, '/global_data_goto'],'GotoTag',['gdata_',str]);
      | 
      | 
      | clear h hblock str
      settings: NameChangeFcn=|
      | h      = get_param(gcb,'handle');   % Get block handle
      | hblock = get(h);     % Parse out handles structure
      | 
      | str = [hblock.Path(numel(bdroot)+2:end), hblock.Name];
      | str(~ismember(str,['A':'Z' 'a':'z' '0':'9' '_'])) = '';
      | set_param([gcb, '/global_data_goto'],'GotoTag',['gdata_',str]);
      | 
      | 
      | clear h hblock str
      mask Display: text(0.25,0.5,'Data Sink')
  Gain : Gain  Gain=1000
  Integrator1 : Integrator  InitialCondition=T_initial
  Scope : Scope
  Sink1 : Subsystem  LoadFcn=rev_comms_sink();  InitFcn=rev_comms_sink();  mask(Sink){}
      mask help: Used for sending data to the upstream component.
      settings: CopyFcn=rev_comms_sink();  NameChangeFcn=rev_comms_sink();
      mask Display: text(0.25,0.5,'Sink')
  Source1 : Subsystem  mask(Source){}
      mask help: Used for receiving data from the downstream component.
      mask init:
      | n_src = gcb;
      | n_src = str2num(n_src(end));
      | try
      |     rev_comms_source(n_src);
      | catch
      | 
      | end
      mask Display: text(0.25,0.5,'Source')
  Source2 : Subsystem  mask(Source){}
      mask help: Used for receiving data from the downstream component.
      mask init:
      | n_src = gcb;
      | n_src = str2num(n_src(end));
      | try
      |     rev_comms_source(n_src);
      | catch
      | 
      | end
      mask Display: text(0.25,0.5,'Source')
  Terminator : Terminator
  Thermal : MATLAB Function  TreatAsAtomicUnit=on
  Voltage : MATLAB Function  TreatAsAtomicUnit=on
  Out1 : Outport
  Out2 : Outport  Port=2
  wires:
  Source2/1(Out1) -> Gain/1
  Voltage/2(Q) -> Scope/1, [Q]
  [I_out] -> Voltage/3(I_out)
  [T] -> Bus Creator2/3  "Temperature [C]"
  [I_in] -> Bus Creator2/1  "Current In [A]"
  [V_out] -> Bus Creator2/2  "Voltage Out [V]"
  Bus Creator2/1 -> Data_Sink/1(" ")
  Thermal/1(T_dot) -> Integrator1/1
  Integrator1/1 -> [T]
  [Q] -> Thermal/1(Q)
  [Q_sink] -> Thermal/2(Q_sink)
  In3/1 -> Current/3(s), Voltage/5(s)
  In2/1 -> Current/2(D), Voltage/4(D)
  Current/1(I_in) -> [I_in], Voltage/2(I_in)
  [I_out] -> Current/1(I_out)
  Voltage/1(V_out) -> [V_out]
  [V_in] -> Voltage/1(V_in)
  [I_out] -> Bus Creator3/1  "current"
  Source1/1(Out1) -> [I_out]
  Bus Selector1/1 -> Terminator/1  "<current>"
  Bus Selector1/2 -> [V_in]  "<voltage>"
  [V_out] -> Bus Creator3/2  "voltage"
  In1/1 -> Bus Selector1/1  "electric"
  Bus Creator3/1 -> Out1/1
  [I_in] -> Sink1/1(In1)
  Bus Creator1/1 -> Out2/1
  [T] -> Bus Creator1/2  "Temp"
  [Q_sink] -> Bus Creator1/1  "Q_kW"
  Gain/1 -> [Q_sink]

== system TestbedModel_v6/Data Manager ==
  Bus Creator : BusCreator  Inputs=1
  Bus Selector1 : BusSelector  OutputSignals=Speed [rad_s]
  SubSystem1 : Subsystem
  Data : Outport
  wires:
  Bus Creator/1 -> Data/1
  [gdata_ShaftData_Sink] -> Bus Selector1/1  "Shaft/Speed [rad_s]"
  Bus Selector1/1 -> SubSystem1/1(Rename)  "<Speed [rad_s]>"
  SubSystem1/1(Bus) -> Bus Creator/1  "Shaft/Speed [rad_s]"

== system TestbedModel_v6/Data Manager1 ==
  Bus Creator : BusCreator  Inputs=1
  Bus Selector1 : BusSelector  OutputSignals=Current In [A]
  SubSystem1 : Subsystem
  Data : Outport
  wires:
  Bus Creator/1 -> Data/1
  [gdata_ConverterData_Sink] -> Bus Selector1/1  "Converter/Current In [A]"
  Bus Selector1/1 -> SubSystem1/1(Rename)  "<Current In [A]>"
  SubSystem1/1(Bus) -> Bus Creator/1  "Converter/Current In [A]"

== system TestbedModel_v6/Data Manager10 ==
  Bus Creator : BusCreator  Inputs=1
  Bus Selector1 : BusSelector  OutputSignals=Current In [A]
  SubSystem1 : Subsystem
  Data : Outport
  wires:
  Bus Creator/1 -> Data/1
  [gdata_Converter1Data_Sink] -> Bus Selector1/1  "Converter1/Current In [A]"
  Bus Selector1/1 -> SubSystem1/1(Rename)  "<Current In [A]>"
  SubSystem1/1(Bus) -> Bus Creator/1  "Converter1/Current In [A]"

== system TestbedModel_v6/Data Manager11 ==
  Bus Creator : BusCreator  Inputs=1
  Bus Selector1 : BusSelector  OutputSignals=Torque [Nm]
  SubSystem1 : Subsystem
  Data : Outport
  wires:
  Bus Creator/1 -> Data/1
  [gdata_Motor1Data_Sink] -> Bus Selector1/1  "Motor1/Torque [Nm]"
  Bus Selector1/1 -> SubSystem1/1(Rename)  "<Torque [Nm]>"
  SubSystem1/1(Bus) -> Bus Creator/1  "Motor1/Torque [Nm]"

== system TestbedModel_v6/Data Manager12 ==
  Bus Creator : BusCreator  Inputs=1
  Bus Selector1 : BusSelector  OutputSignals=Load Torque [Nm]
  SubSystem1 : Subsystem
  Data : Outport
  wires:
  Bus Creator/1 -> Data/1
  [gdata_AirVehicleData_Sink] -> Bus Selector1/1  "Air Vehicle/Load Torque [Nm]"
  Bus Selector1/1 -> SubSystem1/1(Rename)  "<Load Torque [Nm]>"
  SubSystem1/1(Bus) -> Bus Creator/1  "Air Vehicle/Load Torque [Nm]"

== system TestbedModel_v6/Data Manager13 ==
  Bus Creator : BusCreator  Inputs=1
  Bus Selector1 : BusSelector  OutputSignals=Voltage [V]
  SubSystem1 : Subsystem
  Data : Outport
  wires:
  Bus Creator/1 -> Data/1
  [gdata_Capacitor1Data_Sink] -> Bus Selector1/1  "Capacitor1/Voltage [V]"
  Bus Selector1/1 -> SubSystem1/1(Rename)  "<Voltage [V]>"
  SubSystem1/1(Bus) -> Bus Creator/1  "Capacitor1/Voltage [V]"

== system TestbedModel_v6/Data Manager14 ==
  Bus Creator : BusCreator  Inputs=1
  Bus Selector1 : BusSelector  OutputSignals=SOC [-]
  SubSystem1 : Subsystem
  Data : Outport
  wires:
  Bus Creator/1 -> Data/1
  [gdata_BatteryData_Sink] -> Bus Selector1/1  "Battery/SOC [-]"
  Bus Selector1/1 -> SubSystem1/1(Rename)  "<SOC [-]>"
  SubSystem1/1(Bus) -> Bus Creator/1  "Battery/SOC [-]"

== system TestbedModel_v6/Data Manager15 ==
  Bus Creator : BusCreator  Inputs=2
  Bus Selector1 : BusSelector  OutputSignals=SOC [-]
  Bus Selector2 : BusSelector  OutputSignals=Current [A]
  SubSystem1 : Subsystem
  SubSystem2 : Subsystem
  Data : Outport
  wires:
  Bus Creator/1 -> Data/1
  [gdata_BatteryData_Sink] -> Bus Selector1/1  "Battery/SOC [-]"
  Bus Selector1/1 -> SubSystem1/1(Rename)  "<SOC [-]>"
  SubSystem1/1(Bus) -> Bus Creator/1  "Battery/SOC [-]"
  [gdata_BatteryData_Sink] -> Bus Selector2/1  "Battery/Current [A]"
  Bus Selector2/1 -> SubSystem2/1(Rename)  "<Current [A]>"
  SubSystem2/1(Bus) -> Bus Creator/2  "Battery/Current [A]"

== system TestbedModel_v6/Data Manager16 ==
  Bus Creator : BusCreator  Inputs=4
  Bus Selector{1..4} (4 alike) : BusSelector  OutputSignals=Current In [A]
  SubSystem1 : Subsystem
  SubSystem2 : Subsystem
  SubSystem3 : Subsystem
  SubSystem4 : Subsystem
  Data : Outport
  wires:
  Bus Creator/1 -> Data/1
  [gdata_Converter2Data_Sink] -> Bus Selector1/1  "Converter2/Current In [A]"
  Bus Selector1/1 -> SubSystem1/1(Rename)  "<Current In [A]>"
  SubSystem1/1(Bus) -> Bus Creator/1  "Converter2/Current In [A]"
  [gdata_ConverterData_Sink] -> Bus Selector2/1  "Converter/Current In [A]"
  Bus Selector2/1 -> SubSystem2/1(Rename)  "<Current In [A]>"
  SubSystem2/1(Bus) -> Bus Creator/2  "Converter/Current In [A]"
  [gdata_Converter1Data_Sink] -> Bus Selector3/1  "Converter1/Current In [A]"
  Bus Selector3/1 -> SubSystem3/1(Rename)  "<Current In [A]>"
  SubSystem3/1(Bus) -> Bus Creator/3  "Converter1/Current In [A]"
  [gdata_Converter3Data_Sink] -> Bus Selector4/1  "Converter3/Current In [A]"
  Bus Selector4/1 -> SubSystem4/1(Rename)  "<Current In [A]>"
  SubSystem4/1(Bus) -> Bus Creator/4  "Converter3/Current In [A]"

== system TestbedModel_v6/Data Manager17 ==
  Bus Creator : BusCreator  Inputs=1
  Bus Selector1 : BusSelector  OutputSignals=Current [A]
  SubSystem1 : Subsystem
  Data : Outport
  wires:
  Bus Creator/1 -> Data/1
  [gdata_BatteryData_Sink] -> Bus Selector1/1  "Battery/Current [A]"
  Bus Selector1/1 -> SubSystem1/1(Rename)  "<Current [A]>"
  SubSystem1/1(Bus) -> Bus Creator/1  "Battery/Current [A]"

== system TestbedModel_v6/Data Manager18 ==
  Bus Creator : BusCreator  Inputs=1
  Bus Selector1 : BusSelector  OutputSignals=Current In [A]
  SubSystem1 : Subsystem
  Data : Outport
  wires:
  Bus Creator/1 -> Data/1
  [gdata_Converter2Data_Sink] -> Bus Selector1/1  "Converter2/Current In [A]"
  Bus Selector1/1 -> SubSystem1/1(Rename)  "<Current In [A]>"
  SubSystem1/1(Bus) -> Bus Creator/1  "Converter2/Current In [A]"

== system TestbedModel_v6/Data Manager19 ==
  Bus Creator : BusCreator  Inputs=2
  Bus Selector1 : BusSelector  OutputSignals=Current In [A]
  Bus Selector2 : BusSelector  OutputSignals=Current In [A]
  SubSystem1 : Subsystem
  SubSystem2 : Subsystem
  Data : Outport
  wires:
  Bus Creator/1 -> Data/1
  [gdata_Converter2Data_Sink] -> Bus Selector1/1  "Converter2/Current In [A]"
  Bus Selector1/1 -> SubSystem1/1(Rename)  "<Current In [A]>"
  SubSystem1/1(Bus) -> Bus Creator/1  "Converter2/Current In [A]"
  [gdata_Converter3Data_Sink] -> Bus Selector2/1  "Converter3/Current In [A]"
  Bus Selector2/1 -> SubSystem2/1(Rename)  "<Current In [A]>"
  SubSystem2/1(Bus) -> Bus Creator/2  "Converter3/Current In [A]"

== system TestbedModel_v6/Data Manager2 ==
  Bus Creator : BusCreator  Inputs=1
  Bus Selector1 : BusSelector  OutputSignals=Current [A]
  SubSystem1 : Subsystem
  Data : Outport
  wires:
  Bus Creator/1 -> Data/1
  [gdata_MotorData_Sink] -> Bus Selector1/1  "Motor/Current [A]"
  Bus Selector1/1 -> SubSystem1/1(Rename)  "<Current [A]>"
  SubSystem1/1(Bus) -> Bus Creator/1  "Motor/Current [A]"

== system TestbedModel_v6/Data Manager20 ==
  Bus Creator : BusCreator  Inputs=1
  Bus Selector1 : BusSelector  OutputSignals=Speed [rad_s]
  SubSystem1 : Subsystem
  Data : Outport
  wires:
  Bus Creator/1 -> Data/1
  [gdata_ShaftData_Sink] -> Bus Selector1/1  "Shaft/Speed [rad_s]"
  Bus Selector1/1 -> SubSystem1/1(Rename)  "<Speed [rad_s]>"
  SubSystem1/1(Bus) -> Bus Creator/1  "Shaft/Speed [rad_s]"

== system TestbedModel_v6/Data Manager21 ==
  Bus Creator : BusCreator  Inputs=1
  Bus Selector1 : BusSelector  OutputSignals=Current [A]
  SubSystem1 : Subsystem
  Data : Outport
  wires:
  Bus Creator/1 -> Data/1
  [gdata_Motor1Data_Sink] -> Bus Selector1/1  "Motor1/Current [A]"
  Bus Selector1/1 -> SubSystem1/1(Rename)  "<Current [A]>"
  SubSystem1/1(Bus) -> Bus Creator/1  "Motor1/Current [A]"

== system TestbedModel_v6/Data Manager22 ==
  Bus Creator : BusCreator  Inputs=1
  Bus Selector1 : BusSelector  OutputSignals=Speed [rad_s]
  SubSystem1 : Subsystem
  Data : Outport
  wires:
  SubSystem1/1(Bus) -> Bus Creator/1  "Shaft/Speed [rad_s]"
  Bus Selector1/1 -> SubSystem1/1(Rename)  "<Speed [rad_s]>"
  [gdata_ShaftData_Sink] -> Bus Selector1/1  "Shaft/Speed [rad_s]"
  Bus Creator/1 -> Data/1
